simulink model "maxpid_frottements_secs"  (Simulink 7.3)
settings: Solver=ode3  StartTime=0.0  StopTime=1  FixedStep=1e-3  RelTol=1e-3
libraries: simulink x1
settings Model: Creator=Renaud MERLE  LastModifiedBy=Renaud

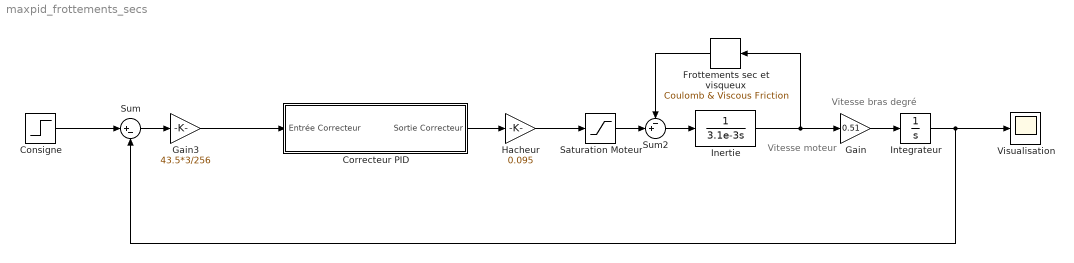
== system maxpid_frottements_secs ==
  note: Vitesse
      | moteur
  note: Vitesse
      | bras degré
  Consigne : Step  Time=0  After=30  SampleTime=0
  Correcteur PID : Subsystem
  Frottements sec et visqueux : simulink/Discontinuities/Coulomb & Viscous Friction  SystemSampleTime=-1  offset=1.5  gain=.075
  Gain : Gain  Gain=0.51  ParameterDataType=fixdt(1, 16)  ParameterScaling=2^0  OutDataType=fixdt(1, 16)  OutScaling=2^0
  Gain3 : Gain  Gain=43.5*3/256  ParameterDataType=fixdt(1, 16)  ParameterScaling=2^0  OutDataType=fixdt(1, 16)  OutScaling=2^0
  Hacheur : Gain  Gain=0.095  ParameterDataType=fixdt(1, 16)  ParameterScaling=2^0  OutDataType=fixdt(1, 16)  OutScaling=2^0
  Inertie : TransferFcn  Denominator=[3.1e-3 0]
  Integrateur : Integrator
  Saturation Moteur : Saturate  UpperLimit=25  LowerLimit=-25  OutDataType=fixdt(1, 16)  OutScaling=2^0
  Sum : Sum  Inputs=|+-  OutDataType=fixdt(1, 16)  OutScaling=2^0
  Sum2 : Sum  Inputs=-+|  OutDataType=fixdt(1, 16)  OutScaling=2^0
  Visualisation : Scope
  wires:
  Consigne/1 -> Sum/1
  Sum/1 -> Gain3/1
  Gain/1 -> Integrateur/1
  Correcteur PID/1(Sortie Correcteur) -> Hacheur/1
  Integrateur/1 -> Sum/2, Visualisation/1
  Hacheur/1 -> Saturation Moteur/1
  Inertie/1 -> Gain/1, Frottements sec et visqueux/1
  Saturation Moteur/1 -> Sum2/2
  Sum2/1 -> Inertie/1
  Gain3/1 -> Correcteur PID/1(Entrée Correcteur)
  Frottements sec et visqueux/1 -> Sum2/1

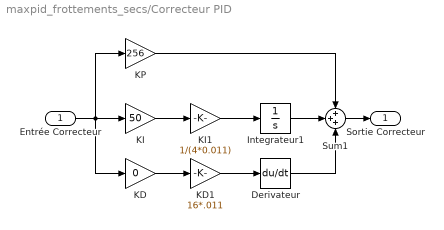
== system maxpid_frottements_secs/Correcteur PID ==
  Entrée Correcteur : Inport
  Derivateur : Derivative
  Integrateur1 : Integrator
  KD : Gain  Gain=0  ParameterDataType=fixdt(1, 16)  ParameterScaling=2^0  OutDataType=fixdt(1, 16)  OutScaling=2^0
  KD1 : Gain  Gain=16*.011  ParameterDataType=fixdt(1, 16)  ParameterScaling=2^0  OutDataType=fixdt(1, 16)  OutScaling=2^0
  KI : Gain  Gain=50  ParameterDataType=fixdt(1, 16)  ParameterScaling=2^0  OutDataType=fixdt(1, 16)  OutScaling=2^0
  KI1 : Gain  Gain=1/(4*0.011)  ParameterDataType=fixdt(1, 16)  ParameterScaling=2^0  OutDataType=fixdt(1, 16)  OutScaling=2^0
  KP : Gain  Gain=256  ParameterDataType=fixdt(1, 16)  ParameterScaling=2^0  OutDataType=fixdt(1, 16)  OutScaling=2^0
  Sum1 : Sum  Inputs=+++  OutDataType=fixdt(1, 16)  OutScaling=2^0
  Sortie Correcteur : Outport
  wires:
  Entrée Correcteur/1 -> KD/1, KP/1, KI/1
  KP/1 -> Sum1/1
  KI/1 -> KI1/1
  KD/1 -> KD1/1
  Integrateur1/1 -> Sum1/2
  Derivateur/1 -> Sum1/3
  KI1/1 -> Integrateur1/1
  KD1/1 -> Derivateur/1
  Sum1/1 -> Sortie Correcteur/1
